simulink model "fccr_complimentary_filter"  (R2017b)
settings: Solver=FixedStepDiscrete  StartTime=0.0  StopTime=inf  RelTol=1e-3  EnableMultiTasking=on
undefined symbols (not defined in the file): DiscIntNeverNeededParam
libraries: simulink x1, simulink_extras x1, beaglebonebluelib x1
settings Model: SimulationMode=external  ExtModeTrigDuration=200  Creator=pthb3  LastModifiedBy=pthb3
settings SolverCC: PositivePriorityOrder=on
settings DataIOCC: InspectSignalLogs=on
settings OptimizationCC: PassReuseOutputArgsAs=Individual arguments  MaxStackSize=64
settings DebuggingCC: ParameterTunabilityLossMsg=error
settings HardwareCC: ProdBitPerPointer=32  ProdBitPerSizeT=32  ProdBitPerPtrDiffT=32  ProdLargestAtomicInteger=Long  ProdLargestAtomicFloat=Double  ProdWordSize=32  ProdHWDeviceType=ARM Compatible->ARM Cortex
settings SFSimCC: MATLABDynamicMemAlloc=off
settings RTWCC: SystemTargetFile=ert.tlc  HardwareBoard=Raspberry Pi  TemplateMakefile=ert_default_tmf  GenerateReport=on  Toolchain=GNU GCC Raspberry Pi  IncludeHyperlinkInReport=on  GenerateTraceInfo=on  GenerateTraceReport=on  GenerateTraceReportSl=on  GenerateTraceReportSf=on  GenerateTraceReportEml=on
settings CodeAppCC: ForceParamTrailComments=on  IgnoreCustomStorageClasses=off  OperatorAnnotations=on  SimulinkDataObjDesc=on  SFDataObjDesc=on  InsertBlockDesc=on
settings ERTTargetCC: SupportVariableSizeSignals=on

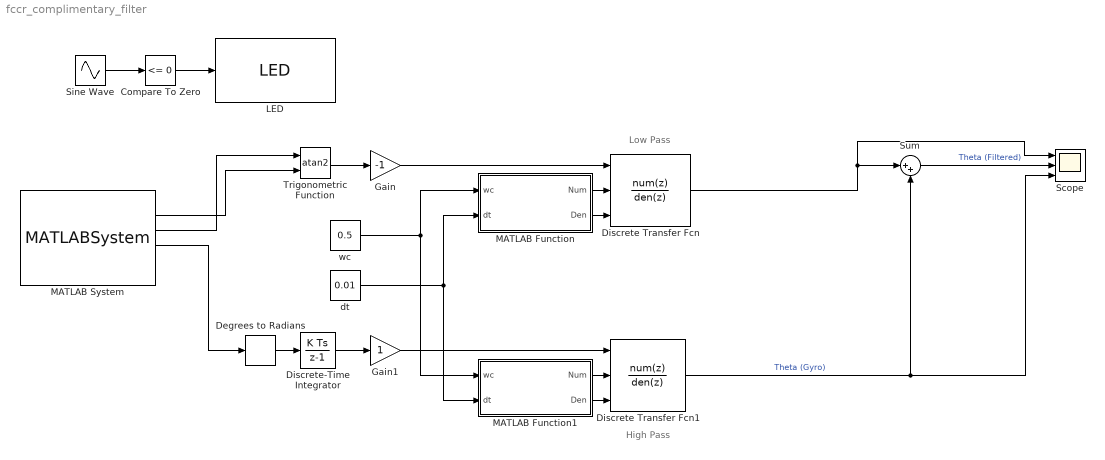
== system fccr_complimentary_filter ==
  note: High Pass
  note: Low Pass
  Compare To Zero : simulink/Logic and Bit Operations/Compare To Zero  relop=<=  OutDataTypeStr=uint8
  Degrees to Radians : simulink_extras/Transformations/Degrees to Radians
  Discrete Transfer Fcn : DiscreteTransferFcn  NumeratorSource=Input port  DenominatorSource=Input port  Denominator=[1]  a0EqualsOne=on
      settings: InputPortMap=u0,p1,p3
  Discrete Transfer Fcn1 : DiscreteTransferFcn  NumeratorSource=Input port  DenominatorSource=Input port  Denominator=[1]  a0EqualsOne=on
      settings: InputPortMap=u0,p1,p3
  Discrete-Time Integrator : DiscreteIntegrator  InitialConditionSetting=State (most efficient)  SampleTime=-1  ICPrevOutput=DiscIntNeverNeededParam  ICPrevScaledInput=DiscIntNeverNeededParam
  Gain : Gain  Gain=-1
  Gain1 : Gain
  LED : beaglebonebluelib/LED  LED=Green
  MATLAB Function : MATLAB Function  TreatAsAtomicUnit=on
  MATLAB Function1 : MATLAB Function  TreatAsAtomicUnit=on
  MATLAB System : MATLABSystem  System=beagleboneblue.fccr_bbblueIMU  SampleTime=0.01
      mask Type: beagleboneblue.fccr_bbblueIMU
      mask Display:
      | color('white');
      | plot([100,100,100,100]*1,[100,100,100,100]*1);
      | plot([100,100,100,100]*0,[100,100,100,100]*0);
      | color('blue');
      | text(100, 92, ' BB BLUE ', 'horizontalAlignment', 'right');
      | color('black');
      | text(52,52,' IMU','horizontalAlignment','center');
      | color('black');
  Scope : Scope  NumInputPorts=3
  Sine Wave : Sin  SineType=Sample based  Frequency=3.14  SampleTime=0.1
  Sum : Sum  Inputs=|++
  Trigonometric Function : Trigonometry  Operator=atan2
  dt : Constant  Value=0.01
  wc : Constant  Value=0.5
  wires:
  Sine Wave/1 -> Compare To Zero/1
  Compare To Zero/1 -> LED/1
  MATLAB System/3 -> Trigonometric Function/1
  MATLAB System/2 -> Trigonometric Function/2
  Trigonometric Function/1 -> Gain/1
  MATLAB System/4 -> Degrees to Radians/1
  Discrete-Time Integrator/1 -> Gain1/1
  Discrete Transfer Fcn1/1 -> Sum/2, Scope/3  "Theta (Gyro)"
  Degrees to Radians/1 -> Discrete-Time Integrator/1
  Sum/1 -> Scope/2  "Theta (Filtered)"
  Gain1/1 -> Discrete Transfer Fcn1/1
  Gain/1 -> Discrete Transfer Fcn/1
  Discrete Transfer Fcn/1 -> Scope/1, Sum/1
  MATLAB Function/1(Num) -> Discrete Transfer Fcn/2
  MATLAB Function/2(Den) -> Discrete Transfer Fcn/3
  MATLAB Function1/1(Num) -> Discrete Transfer Fcn1/2
  MATLAB Function1/2(Den) -> Discrete Transfer Fcn1/3
  wc/1 -> MATLAB Function1/1(wc), MATLAB Function/1(wc)
  dt/1 -> MATLAB Function1/2(dt), MATLAB Function/2(dt)

== matlab function fccr_complimentary_filter/MATLAB Function1 ==
  data: wc input; Num output; dt input; Den output
function [Num, Den] = first_order_hp(wc,dt)
%#codegen
Num = [1 -1];
Den = [1 (wc*dt - 1)];

== matlab function fccr_complimentary_filter/MATLAB Function ==
  data: wc input; Num output; dt input; Den output
function [Num, Den] = first_order_lp(wc,dt)
%#codegen
Num = [0 wc*dt];
Den = [1 (wc*dt - 1)];
